simulink model "Feedback_Control_Template"  (R2024b)
settings: Solver=VariableStepAuto  StartTime=0.0  StopTime=10.0  RelTol=1e-3
settings Model: Creator=sh2323  LastModifiedBy=sh2323

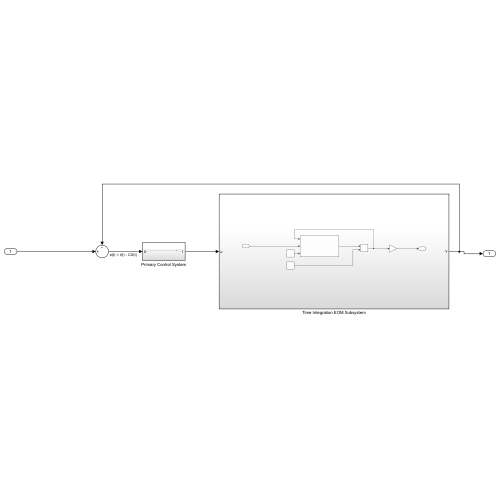
[thumbnail: Simulink's stored preview of the top-level diagram]
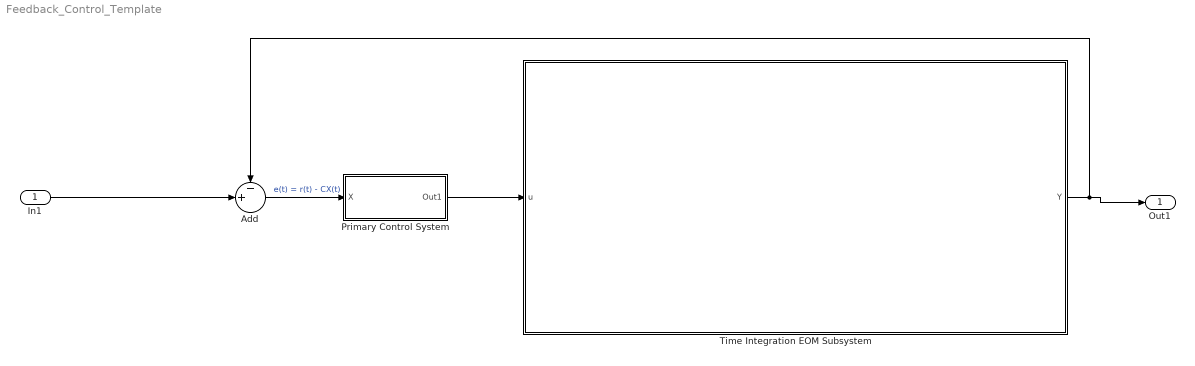
== system Feedback_Control_Template ==
  In1 : Inport
  Add : Sum  Inputs=-+|
  Primary Control System : Subsystem
  Time Integration EOM Subsystem : Subsystem
  Out1 : Outport
  wires:
  Primary Control System/1(Out1) -> Time Integration EOM Subsystem/1(u)
  Add/1 -> Primary Control System/1(X)  "e(t) = r(t) - CX(t)"
  Time Integration EOM Subsystem/1(Y) -> Add/1, Out1/1
  In1/1 -> Add/2

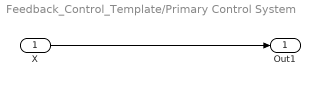
== system Feedback_Control_Template/Primary Control System ==
  X : Inport
  Out1 : Outport
  wires:
  X/1 -> Out1/1

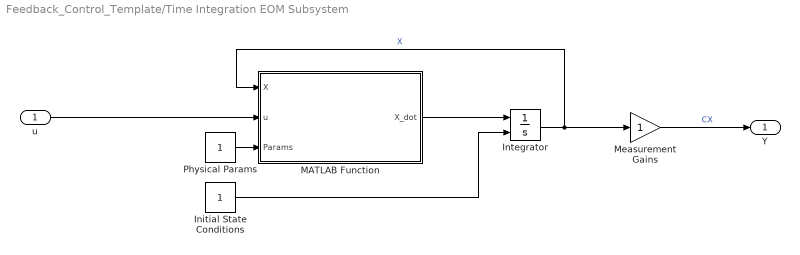
== system Feedback_Control_Template/Time Integration EOM Subsystem ==
  u : Inport
  Initial State Conditions : Constant
  Integrator : Integrator  InitialConditionSource=external
  MATLAB Function : MATLAB Function  TreatAsAtomicUnit=on
  Measurement Gains : Gain
  Physical Params : Constant
  Y : Outport
  wires:
  MATLAB Function/1(X_dot) -> Integrator/1
  Integrator/1 -> Measurement Gains/1, MATLAB Function/1(X)  "X"
  Physical Params/1 -> MATLAB Function/3(Params)
  Initial State Conditions/1 -> Integrator/2
  Measurement Gains/1 -> Y/1  "CX"
  u/1 -> MATLAB Function/2(u)

== matlab function Feedback_Control_Template/Time Integration EOM Subsystem/MATLAB Function ==
  data: X input; u input; X_dot output; Params input
function X_dot = EOM(X,u,Params)

y = u;
